simulink model "lab03"  (Simulink 9.2)
settings: Solver=ode45  StartTime=0.0  StopTime=0.15  RelTol=1e-3  EnableMultiTasking=on
values from neighbouring files (symbols this model uses):
  Ja = 0.00002    (= 2e-05)    [lab03.m]
  Ke = 0.057    [lab03.m]
  Km = 0.057    [lab03.m]
  La = 0.004    [lab03.m]
  M = Mnom*2*i1/(Nm-1); M1(i)=M    [lab03.m]
  Ra = 4.0    (= 4)    [lab03.m]
  T = 0.001    [lab03.m]
  U = 1.25*2*j1/(Nu-1); U1(j)=U    [lab03.m]
  Umax = Unom    (= 24)    [lab03.m]
settings Model: Creator=PC  LastModifiedBy=PC  ExtModeTrigMode=oneshot  ExtModeArmWhenConnect=off
settings DataIOCC: LimitDataPoints=off  SignalLoggingName=sigsOut
settings OptimizationCC: BooleanDataType=off  LifeSpan=auto
settings DebuggingCC: SaveWithParameterizedLinksMsg=none  SignalResolutionControl=TryResolveAllWithWarning  MultiTaskDSMMsg=warning  MultiTaskCondExecSysMsg=none  FcnCallInpInsideContextMsg=error  StateNameClashWarn=none  SFUnexpectedBacktrackingDiag=error  SFNoUnconditionalDefaultTransitionDiag=error  SFExecutionAtInitializationDiag=warning
settings HardwareCC: TargetUnknown=on
settings SFSimCC: SimUseLocalCustomCode=on
settings RTWCC: RTWUseLocalCustomCode=on
settings CodeAppCC: StateflowObjectComments=off
settings GRTTargetCC: TargetLangStandard=C99 (ISO)  GeneratePreprocessorConditionals=Use local settings
settings ConfigComp: CovExternalEMLEnable=on

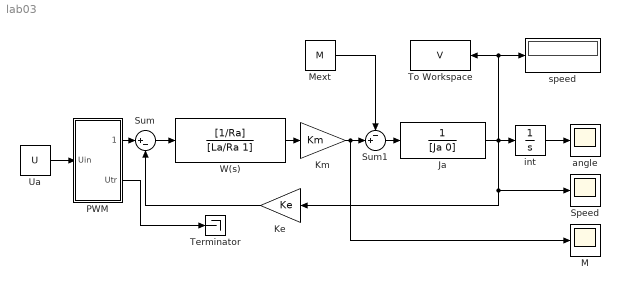
== system lab03 ==
  Ja : TransferFcn  Denominator=[Ja 0]
  Ke : Gain  Gain=Ke  SaturateOnIntegerOverflow=on  OutDataTypeStr=Inherit: Same as input  ParamDataTypeStr=Inherit: Same as input
  Km : Gain  Gain=Km  SaturateOnIntegerOverflow=on  OutDataTypeStr=Inherit: Same as input  ParamDataTypeStr=Inherit: Same as input
  M : Scope
  Mext : Constant  Value=M
  PWM : Subsystem
  Speed : Scope
  Sum : Sum  Inputs=|+-  SaturateOnIntegerOverflow=on  InputSameDT=on  OutDataTypeStr=Inherit: Same as first input
  Sum1 : Sum  Inputs=-+|  SaturateOnIntegerOverflow=on  InputSameDT=on  OutDataTypeStr=Inherit: Same as first input
  Terminator : Terminator
  To Workspace : ToWorkspace  VariableName=V  SampleTime=-1
  Ua : Constant  Value=U
  W(s) : TransferFcn  Numerator=[1/Ra]  Denominator=[La/Ra 1]
  angle : Scope
  int : Integrator
  speed : Display
  wires:
  Sum/1 -> W(s)/1
  W(s)/1 -> Km/1
  Mext/1 -> Sum1/1
  Ke/1 -> Sum/2
  Sum1/1 -> Ja/1
  Ja/1 -> Ke/1, Speed/1, int/1, To Workspace/1, speed/1
  int/1 -> angle/1
  Km/1 -> Sum1/2, M/1
  Ua/1 -> PWM/1(Uin)
  PWM/1(Uout) -> Sum/1
  PWM/2(Utr) -> Terminator/1

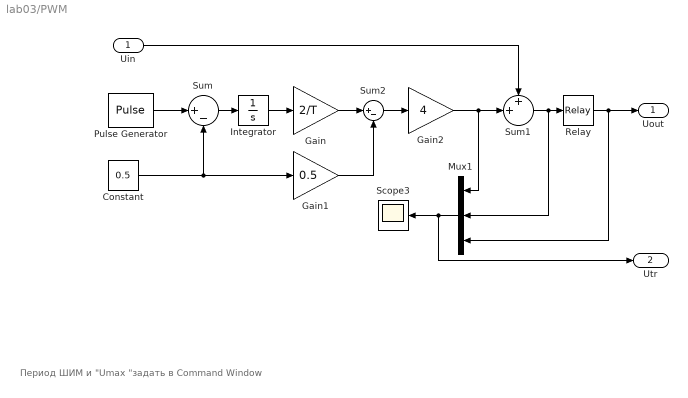
== system lab03/PWM ==
  note: Период ШИМ и "Umax "задать в Command Window
  Uin : Inport
  Constant : Constant  Value=0.5
  Gain : Gain  Gain=2/T  SaturateOnIntegerOverflow=on  OutDataTypeStr=Inherit: Same as input  ParamDataTypeStr=Inherit: Same as input
  Gain1 : Gain  Gain=0.5  SaturateOnIntegerOverflow=on  OutDataTypeStr=Inherit: Same as input  ParamDataTypeStr=Inherit: Same as input
  Gain2 : Gain  Gain=4  SaturateOnIntegerOverflow=on  OutDataTypeStr=Inherit: Same as input  ParamDataTypeStr=Inherit: Same as input
  Integrator : Integrator
  Mux1 : Mux  Inputs=3
  Pulse Generator : DiscretePulseGenerator  PulseType=Time based  Period=T  PulseWidth=50  VectorParams1D=off
  Relay : Relay  OnSwitchValue=0  OffSwitchValue=0  OnOutputValue=Umax  OffOutputValue=-Umax
  Scope3 : Scope
  Sum : Sum  Inputs=|+-  SaturateOnIntegerOverflow=on
  Sum1 : Sum  Inputs=++|  SaturateOnIntegerOverflow=on
  Sum2 : Sum  Inputs=|+-  SaturateOnIntegerOverflow=on
  Uout : Outport
  Utr : Outport  Port=2
  wires:
  Pulse Generator/1 -> Sum/1
  Constant/1 -> Sum/2, Gain1/1
  Sum/1 -> Integrator/1
  Integrator/1 -> Gain/1
  Gain/1 -> Sum2/1
  Relay/1 -> Uout/1, Mux1/3
  Gain1/1 -> Sum2/2
  Sum2/1 -> Gain2/1
  Uin/1 -> Sum1/1
  Gain2/1 -> Sum1/2, Mux1/1
  Mux1/1 -> Scope3/1, Utr/1
  Sum1/1 -> Relay/1, Mux1/2
